simulink library "custom_PIDs_1DOF_w_reset"  (R2016b)
settings: Solver=VariableStepAuto  StartTime=0.0  StopTime=10.0  RelTol=1e-3
settings Model: Creator=Flyart  LastModifiedBy=Flyart

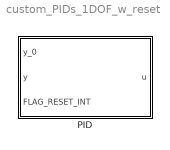
== system custom_PIDs_1DOF_w_reset ==
  PID : Subsystem  mask{Kf=0, Kp=0, Ki=0, Kd=0, N=1, min_u=0, max_u=0, ts=0.01}

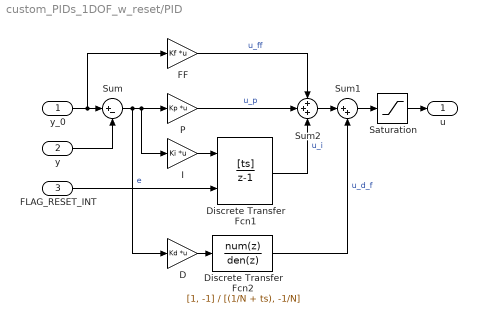
== system custom_PIDs_1DOF_w_reset/PID ==
  y_0 : Inport
  y : Inport  Port=2
  FLAG_RESET_INT : Inport  Port=3
  D : Gain  Gain=Kd  Multiplication=Matrix(K*u)
  Discrete Transfer Fcn1 : DiscreteTransferFcn  Numerator=[ts]  Denominator=[1, -1]  ExternalReset=Level hold  SampleTime=ts
      settings: InputPortMap=u0,r7
  Discrete Transfer Fcn2 : DiscreteTransferFcn  Numerator=[1, -1]  Denominator=[(1/N + ts), -1/N]  SampleTime=ts
  FF : Gain  Gain=Kf  Multiplication=Matrix(K*u)
  I : Gain  Gain=Ki  Multiplication=Matrix(K*u)
  P : Gain  Gain=Kp  Multiplication=Matrix(K*u)
  Saturation : Saturate  UpperLimit=max_u  LowerLimit=min_u
  Sum : Sum  Inputs=|+-
  Sum1 : Sum  Inputs=|++
  Sum2 : Sum  Inputs=+++
  u : Outport
  wires:
  Sum/1 -> D/1, I/1, P/1  "e"
  Sum1/1 -> Saturation/1
  Sum2/1 -> Sum1/1
  y_0/1 -> FF/1, Sum/1
  I/1 -> Discrete Transfer Fcn1/1
  D/1 -> Discrete Transfer Fcn2/1
  y/1 -> Sum/2
  P/1 -> Sum2/2  "u_p"
  Discrete Transfer Fcn1/1 -> Sum2/3  "u_i"
  FF/1 -> Sum2/1  "u_ff"
  Saturation/1 -> u/1
  Discrete Transfer Fcn2/1 -> Sum1/2  "u_d_f"
  FLAG_RESET_INT/1 -> Discrete Transfer Fcn1/2
